simulink model "Q2_full_bridge_converter"  (R2016a)
settings: Solver=VariableStepAuto  StartTime=0.0  StopTime=15e-3  MaxStep=1e-4  RelTol=1e-3
libraries: powerlib x17, powerlib_meascontrol x1, dspstat3 x1
settings Model: Creator=syf  LastModifiedBy=DELL
settings SimscapeCC: SimscapeNormalizeSystem=off

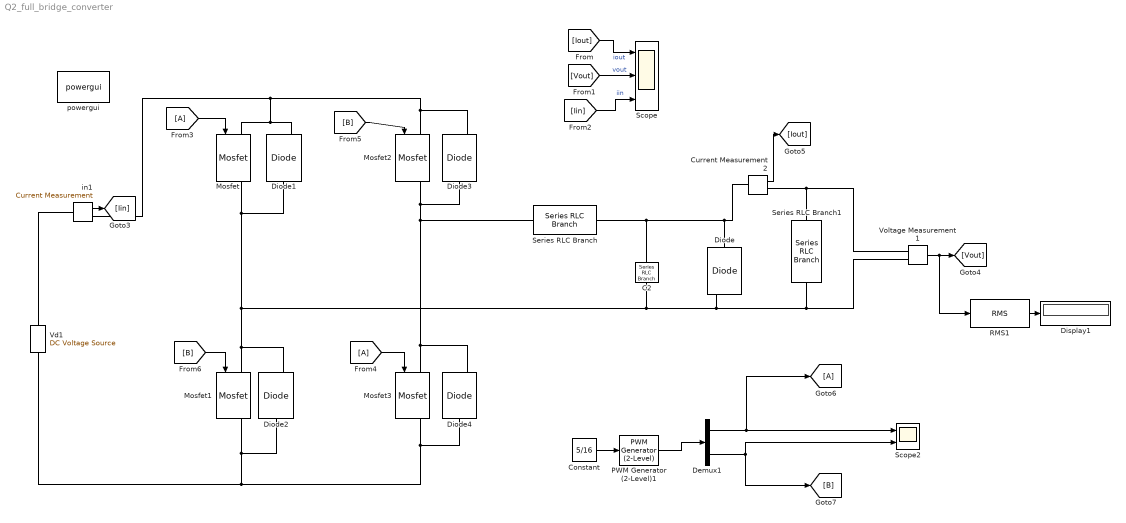
== system Q2_full_bridge_converter ==
  C2 : powerlib/Elements/Series RLC Branch  LConnTagsString=__new0  RConnTagsString=__new0  BranchType=C  Resistance=1  Inductance=1e-3  SetiL0=off  InitialCurrent=0  Capacitance=470e-6  Setx0=off  InitialVoltage=25  Measurements=None
  Constant : Constant  Value=5/16
  Current Measurement2 : powerlib/Measurements/Current Measurement  PhasorSimulation=off  OutputType=Complex  PSBequivalent=0
  Demux1 : Demux  Outputs=2
  Diode : powerlib/Power Electronics/Diode  Ron=0.001  Lon=0  Vf=15  IC=0  UseSnubber=0  Rs=500  Cs=250e-9  Measurements=on
  Diode{1..4} (4 alike) : powerlib/Power Electronics/Diode  Ron=0.001  Lon=0  Vf=0.8  IC=0  UseSnubber=off  Rs=500  Cs=250e-9  Measurements=on
  Display1 : Display
  Mosfet{,1..3} (4 alike) : powerlib/Power Electronics/Mosfet  Ron=0.1  Lon=0  Rd=0.01  Vfd=0  IC=0  Rs=1e5  Cs=inf  Measurements=on
  PWM Generator (2-Level)1 : powerlib_meascontrol/Pulse & Signal Generators/PWM Generator (2-Level)  ModulatorType=Single-phase half-bridge (2 pulses)  ModulatorMode=Unsynchronized  Fc=20e3  Pc=0  nF=27  MinMax="[ 0  1 ]"  SamplingTechnique=Natural  ModulatingSignals=off  m=5/16  Freq=60  Phase=0  Ts=0  ShowCarrierOutport=off
  RMS1 : dspstat3/RMS  run=off  directionMode=Each column  dimension=1  InputProcessing=Columns as channels (frame based)  reset_popup=None
  Scope : Scope  NumInputPorts=3
  Scope2 : Scope  NumInputPorts=2
  Series RLC Branch : powerlib/Elements/Series RLC Branch  LConnTagsString=__new0  RConnTagsString=__new0  BranchType=L  Resistance=1  Inductance=5600e-6  SetiL0=off  InitialCurrent=0  Capacitance=1e-6  Setx0=off  InitialVoltage=0  Measurements=None
  Series RLC Branch1 : powerlib/Elements/Series RLC Branch  LConnTagsString=__new0  RConnTagsString=__new0  BranchType=RL  Resistance=1.2  Inductance=3e-3  SetiL0=off  InitialCurrent=0  Capacitance=1e-6  Setx0=off  InitialVoltage=0  Measurements=None
  Vd1 : powerlib/Electrical Sources/DC Voltage Source  Amplitude=48  Measurements=None
  Voltage Measurement1 : powerlib/Measurements/Voltage Measurement  PhasorSimulation=off  OutputType=Complex  PSBequivalent=0
  in1 : powerlib/Measurements/Current Measurement  PhasorSimulation=off  OutputType=Complex  PSBequivalent=0
  powergui : powerlib/powergui  Priority=1  SimulationMode=Continuous  SampleTime=50e-6  frequency=60  Iterations=250  frequencyindice=0  Pbase=100e6  ErrMax=1e-4  UnitsV=kV  UnitsW=MW  buscounter=0  FunctionMessages=off  echomessages=off  EnableUseOfTLC=off  CurrentSourceSwitches=off  DisableSnubberDevices=off  DisableRonSwitches=off  DisableVfSwitches=off  DisplayEquations=off  SolverType=Tustin/Backward Euler (TBE)  Interpol=off  ExternalGateDelay=off  methode=off  Ts=100  x0status=blocks  SPID=on  SwTol=0  HookPort=off  RestoreLinks=warning  ResistiveCurrentMeasurement=off  Frange=[0:2:500]  Ylog=off  Xlog=on  ShowGrid=off  save=off  variable=ZData  structure=0  ZoomFFT=off  StartTime=0.0  cycles=1  DisplayStyle=1  fundamental=60  FreqAxis=off  MaxFrequency=1000  frequencyindicesteady=1  RmsSteady=1  display=off
  wires:
  [Vout] -> Scope/2  "vout"
  [Iout] -> Scope/1  "iout"
  [Iin] -> Scope/3  "iin"
  in1/1 -> [Iin]
  Voltage Measurement1/1 -> [Vout], RMS1/1
  Current Measurement2/1 -> [Iout]
  RMS1/1 -> Display1/1
  PWM Generator (2-Level)1/1 -> Demux1/1
  Demux1/1 -> Scope2/1, [A]
  Demux1/2 -> [B], Scope2/2
  Constant/1 -> PWM Generator (2-Level)1/1
  [A] -> Mosfet/1
  [A] -> Mosfet3/1
  [B] -> Mosfet2/1
  [B] -> Mosfet1/1
  connections:
  Diode1/RConn1 -- in1/RConn1 -- Diode3/RConn1 -- Mosfet2/LConn1 -- Mosfet/LConn1
  Vd1/LConn1 -- Diode4/LConn1 -- Mosfet3/RConn1 -- Diode2/LConn1 -- Mosfet1/RConn1
  in1/LConn1 -- Vd1/RConn1
  Series RLC Branch1/LConn1 -- Current Measurement2/RConn1 -- Voltage Measurement1/LConn1
  Mosfet/RConn1 -- Diode1/LConn1 -- Diode/RConn1 -- Series RLC Branch1/RConn1 -- Voltage Measurement1/LConn2 -- C2/RConn1 -- Diode2/RConn1 -- Mosfet1/LConn1
  Diode4/RConn1 -- Series RLC Branch/LConn1 -- Mosfet2/RConn1 -- Diode3/LConn1 -- Mosfet3/LConn1
  Current Measurement2/LConn1 -- Diode/LConn1 -- Series RLC Branch/RConn1 -- C2/LConn1
